simulink model "gm_inc_enc_v26"  (R2023a)
settings: Solver=FixedStepDiscrete  StartTime=0.0  StopTime=SimulationsDauer  RelTol=1e-3
undefined symbols (not defined in the file or in its folder): CW_CCW_Switch, d_axis_hit_CompareValue, DiscIntNeverNeededParam, f_ISR, IncPerTurn, inital_zero_speed_timeout, n_max, Offset_Position_elec, Offset_Position_mech, OmegaPerOverSampl, Periode, Phase_Delay_A, Phase_Delay_B, PolePair, QuadratureFactor, reciprocal_iterations, T_fpga, T_mech
libraries: hdlmdlgenlib x16, dspsrcs4 x3, dspswit3 x2, spsEdgeDetectorLib x2, simulink_extras x1
(part 1 of 3)
settings Model: Creator=Wendel_ELSYS  LastModifiedBy=ts
settings SolverCC: ConcurrentTasks=on  AlgebraicLoopSolver=TrustRegion  MinimalZcImpactIntegration=on
settings DataIOCC: LimitDataPoints=on  SaveFormat=Array
settings OptimizationCC: BlockReduction=off  ConditionallyExecuteInputs=off  DefaultParameterBehavior=Inlined  InheritOutputTypeSmallerThanSingle=on  ReuseModelBlockBuffer=off  LifeSpan=inf
settings DebuggingCC: ReadBeforeWriteMsg=DisableAll  WriteAfterWriteMsg=DisableAll  WriteAfterReadMsg=DisableAll  AlgebraicLoopMsg=error  InheritedTsInSrcMsg=none  SingleTaskRateTransMsg=error  ParameterOverflowMsg=none  UnconnectedInputMsg=warning  UnconnectedOutputMsg=warning  UnconnectedLineMsg=warning  SFUnexpectedBacktrackingDiag=warning  SFNoUnconditionalDefaultTransitionDiag=warning  SFExecutionAtInitializationDiag=none  ArithmeticOperatorsInVariantConditions=warning
settings HardwareCC: ProdBitPerPointer=32  ProdBitPerSizeT=32  ProdBitPerPtrDiffT=32  ProdLargestAtomicFloat=None  ProdIntDivRoundTo=Undefined  ProdEndianess=Unspecified  ProdWordSize=32  ProdHWDeviceType=ASIC/FPGA->ASIC/FPGA  ProdEqTarget=off
settings ModelReferenceCC: UpdateModelReferenceTargets=IfOutOfDate  EnableRefExpFcnMdlSchedulingChecks=on  PropagateSignalLabelsOutOfModel=off
settings SFSimCC: SFSimEcho=off  SimUseLocalCustomCode=off  CustomCodeUndefinedFunction=UseInterfaceOnly
settings RTWCC: RTWUseLocalCustomCode=off  DLArmComputeVersion=19.05
settings CodeAppCC: StateflowObjectComments=on
settings GRTTargetCC: TargetLangStandard=C89/C90 (ANSI)
settings ConfigComp: CovMetricSettings=dw  CovSaveCumulativeToWorkspaceVar=on  CovSaveSingleToWorkspaceVar=on  CovExternalEMLEnable=off
settings SimscapeCC: SimscapeNormalizeSystem=off

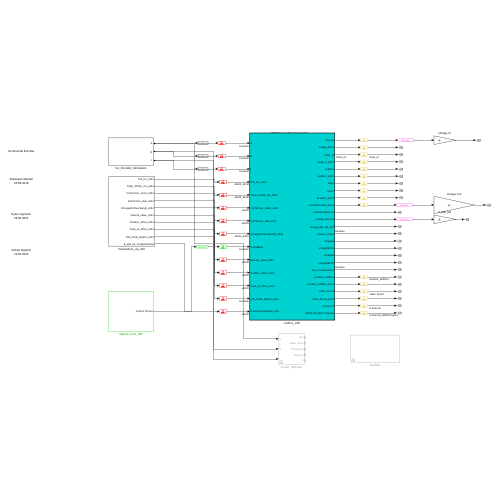
[thumbnail: Simulink's stored preview of the top-level diagram]
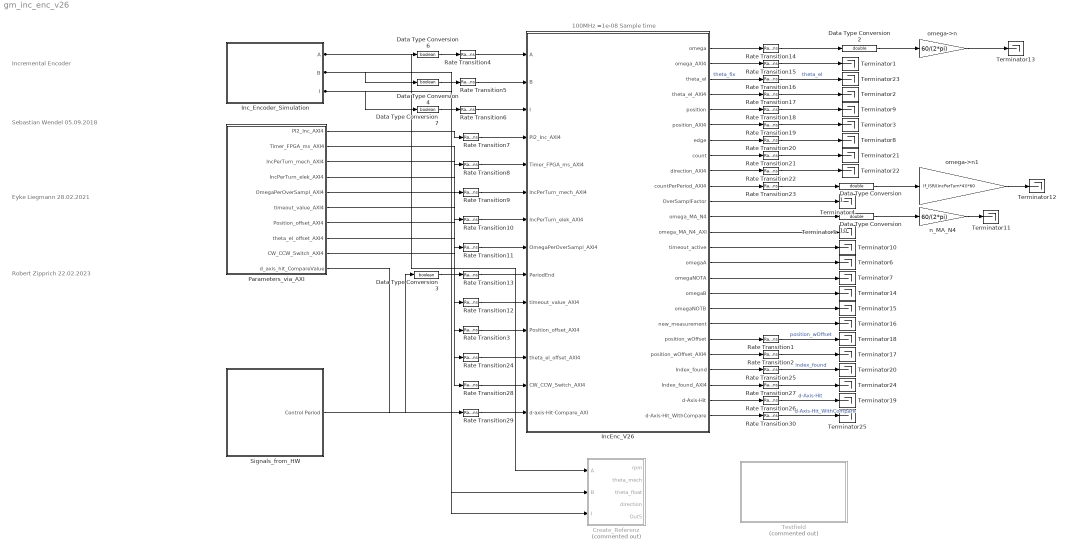
== system gm_inc_enc_v26 ==
  note: Robert Zipprich
      | 22.02.2023
  note: Eyke Liegmann
      | 28.02.2021
  note: Incremental Encoder
  note: Sebastian Wendel
      | 05.09.2018
  note: 100MHz =1e-08 Sample time
  Create_Referenz : Subsystem  Commented=on
  Data Type Conversion1 : DataTypeConversion  OutDataTypeStr=double  SaturateOnIntegerOverflow=off  RndMeth=Floor
  Data Type Conversion10 : DataTypeConversion  OutDataTypeStr=double  SaturateOnIntegerOverflow=off  RndMeth=Floor
  Data Type Conversion2 : DataTypeConversion  OutDataTypeStr=double  SaturateOnIntegerOverflow=off  RndMeth=Floor
  Data Type Conversion{3..4,6..7} (4 alike) : DataTypeConversion  OutDataTypeStr=boolean  SaturateOnIntegerOverflow=off  RndMeth=Floor
  IncEnc_V26 : Subsystem  TreatAsAtomicUnit=on
  Inc_Encoder_Simulation : Subsystem
  Parameters_via_AXI : Subsystem
  Rate Transition{1..2,14..23,25..27,30} (16 alike) : RateTransition  Deterministic=off  OutPortSampleTime=T_mech
  Rate Transition{3..13,24,28..29} (14 alike) : RateTransition  Deterministic=off  OutPortSampleTime=T_fpga
  Signals_from_HW : Subsystem
  Terminator{1..25} (25 alike) : Terminator
  Testfield : Subsystem  Commented=on
  n_MA_N4 : Gain  Gain=60/(2*pi)  OutDataTypeStr=double
  omega->n : Gain  Gain=60/(2*pi)  OutDataTypeStr=double
  omega->n1 : Gain  Gain=(f_ISR/(IncPerTurn*4))*60  OutDataTypeStr=double
  wires:
  Rate Transition30/1 -> Terminator25/1  "d-Axis-Hit_WithCompare"
  IncEnc_V26/25(d-Axis-Hit_WithCompare) -> Rate Transition30/1
  Parameters_via_AXI/10(d_axis_hit_CompareValue) -> Rate Transition29/1
  Rate Transition29/1 -> IncEnc_V26/14(d-axis-Hit-Compare_AXI)
  Parameters_via_AXI/9(CW_CCW_Switch_AXI4) -> Rate Transition28/1
  Rate Transition28/1 -> IncEnc_V26/13(CW_CCW_Switch_AXI4)
  IncEnc_V26/23(Index_found_AXI4) -> Rate Transition27/1
  Rate Transition27/1 -> Terminator24/1
  Rate Transition16/1 -> Terminator23/1  "theta_el"
  Rate Transition21/1 -> Terminator21/1
  Rate Transition22/1 -> Terminator22/1
  IncEnc_V26/24(d-Axis-Hit) -> Rate Transition26/1
  Rate Transition26/1 -> Terminator19/1  "d-Axis-Hit"
  Rate Transition25/1 -> Terminator20/1  "index_found"
  IncEnc_V26/22(Index_found) -> Rate Transition25/1
  Parameters_via_AXI/8(theta_el_offset_AXI4) -> Rate Transition24/1
  Rate Transition24/1 -> IncEnc_V26/12(theta_el_offset_AXI4)
  Parameters_via_AXI/7(Position_offset_AXI4) -> Rate Transition3/1
  Rate Transition3/1 -> IncEnc_V26/11(Position_offset_AXI4)
  IncEnc_V26/20(position_wOffset) -> Rate Transition1/1
  IncEnc_V26/21(position_wOffset_AXI4) -> Rate Transition2/1
  Rate Transition2/1 -> Terminator17/1
  Rate Transition1/1 -> Terminator18/1  "position_wOffset"
  Signals_from_HW/1(Control Period) -> Data Type Conversion3/1
  Inc_Encoder_Simulation/1(A) -> Create_Referenz/1(A), Data Type Conversion6/1
  Inc_Encoder_Simulation/3(I) -> Data Type Conversion7/1, Create_Referenz/3(I)
  Inc_Encoder_Simulation/2(B) -> Data Type Conversion4/1, Create_Referenz/2(B)
  Parameters_via_AXI/6(timeout_value_AXI4) -> Rate Transition12/1
  Parameters_via_AXI/5(OmegaPerOverSampl_AXI4) -> Rate Transition11/1
  Parameters_via_AXI/4(IncPerTurn_elek_AXI4) -> Rate Transition10/1
  Parameters_via_AXI/3(IncPerTurn_mech_AXI4) -> Rate Transition9/1
  Parameters_via_AXI/2(Timer_FPGA_ms_AXI4) -> Rate Transition8/1
  Parameters_via_AXI/1(PI2_Inc_AXI4) -> Rate Transition7/1
  IncEnc_V26/19(new_measurement) -> Terminator16/1
  IncEnc_V26/16(omegaNOTA) -> Terminator7/1
  IncEnc_V26/17(omegaB) -> Terminator14/1
  IncEnc_V26/18(omegaNOTB) -> Terminator15/1
  IncEnc_V26/15(omegaA) -> Terminator6/1
  omega->n1/1 -> Terminator12/1
  n_MA_N4/1 -> Terminator11/1
  Rate Transition18/1 -> Terminator9/1
  Rate Transition20/1 -> Terminator8/1
  IncEnc_V26/14(timeout_active) -> Terminator10/1
  Rate Transition12/1 -> IncEnc_V26/10(timeout_value_AXI4)
  Data Type Conversion10/1 -> n_MA_N4/1
  IncEnc_V26/13(omega_MA_N4_AXI) -> Terminator5/1
  IncEnc_V26/12(omega_MA_N4) -> Data Type Conversion10/1
  IncEnc_V26/11(OverSamplFactor) -> Terminator4/1
  Rate Transition23/1 -> Data Type Conversion1/1
  Rate Transition19/1 -> Terminator3/1
  Rate Transition17/1 -> Terminator2/1
  Rate Transition15/1 -> Terminator1/1
  Rate Transition14/1 -> Data Type Conversion2/1
  Rate Transition13/1 -> IncEnc_V26/9(PeriodEnd)
  Rate Transition11/1 -> IncEnc_V26/8(OmegaPerOverSampl_AXI4)
  Rate Transition10/1 -> IncEnc_V26/7(IncPerTurn_elek_AXI4)
  Rate Transition9/1 -> IncEnc_V26/6(IncPerTurn_mech_AXI4)
  Rate Transition8/1 -> IncEnc_V26/5(Timer_FPGA_ms_AXI4)
  Rate Transition7/1 -> IncEnc_V26/4(PI2_Inc_AXI4)
  Rate Transition6/1 -> IncEnc_V26/3(I)
  Rate Transition5/1 -> IncEnc_V26/2(B)
  Rate Transition4/1 -> IncEnc_V26/1(A)
  IncEnc_V26/6(position_AXI4) -> Rate Transition19/1
  Data Type Conversion3/1 -> Rate Transition13/1
  IncEnc_V26/10(countPerPeriod_AXI4) -> Rate Transition23/1
  Data Type Conversion1/1 -> omega->n1/1
  Data Type Conversion2/1 -> omega->n/1
  omega->n/1 -> Terminator13/1
  IncEnc_V26/2(omega_AXI4) -> Rate Transition15/1
  IncEnc_V26/4(theta_el_AXI4) -> Rate Transition17/1
  IncEnc_V26/5(position) -> Rate Transition18/1
  IncEnc_V26/3(theta_el) -> Rate Transition16/1  "theta_fix"
  IncEnc_V26/8(count) -> Rate Transition21/1
  IncEnc_V26/7(edge) -> Rate Transition20/1
  IncEnc_V26/9(direction_AXI4) -> Rate Transition22/1
  IncEnc_V26/1(omega) -> Rate Transition14/1
  Data Type Conversion7/1 -> Rate Transition6/1
  Data Type Conversion4/1 -> Rate Transition5/1
  Data Type Conversion6/1 -> Rate Transition4/1

== system gm_inc_enc_v26/Create_Referenz ==
  note: Überprüfen der Ausgabe:
      | (1/((Wert in Periodfelt von Counter)*Inkremente))*60
      | z.B. (1/((2.5*0.000001)*5000))*60
  A : Inport
  B : Inport  Port=2
  I : Inport  Port=3
  HardwareTimer_FPGA_in_ms*InCrements1 : Constant  Value=T_mech*IncPerTurn  OutDataTypeStr=double  SampleTime=T_mech
  IncrementalEncoder_Floating : Subsystem  Commented=on
  "daQuadraturEncoder " : Gain  Commented=on  Gain=4
  n_aus_theta : Subsystem  Commented=on  TreatAsAtomicUnit=on
  poles : Constant  Value=PolePair  OutDataTypeStr=uint8  SampleTime=T_mech
  rpm : Outport
  theta_mech : Outport  Port=2
  theta_float : Outport  Port=3
  direction : Outport  Port=4
  Out5 : Outport  Port=5
  wires:
  IncrementalEncoder_Floating/2(theta_mech) -> theta_mech/1
  "daQuadraturEncoder "/1 -> Out5/1
  IncrementalEncoder_Floating/1(rpm) -> rpm/1
  IncrementalEncoder_Floating/4(direction) -> direction/1
  HardwareTimer_FPGA_in_ms*InCrements1/1 -> n_aus_theta/2(T)
  I/1 -> IncrementalEncoder_Floating/3(I)
  poles/1 -> IncrementalEncoder_Floating/4(poles)
  IncrementalEncoder_Floating/3(theta_elec) -> theta_float/1  "theta_float"
  B/1 -> IncrementalEncoder_Floating/2(B)
  A/1 -> n_aus_theta/1(count), IncrementalEncoder_Floating/1(A)
  n_aus_theta/1(rpm) -> "daQuadraturEncoder "/1

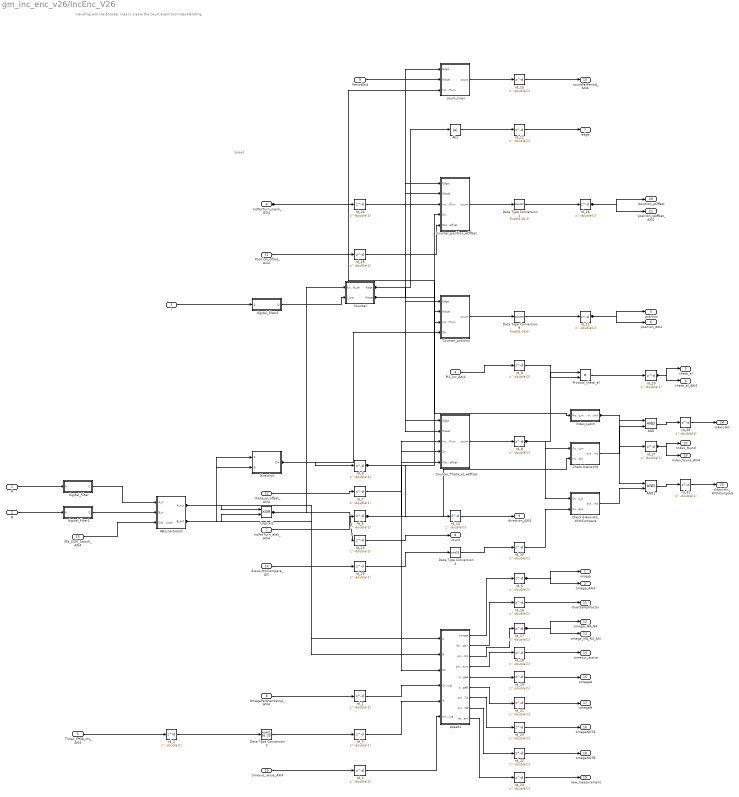
== system gm_inc_enc_v26/IncEnc_V26 ==
  note: Speed
  note: Handling with the Encoder lines to create the Count-Event and Index-Handling
  A : Inport  OutDataTypeStr=boolean  PortDimensions=1  SampleTime=1e-08
  B : Inport  Port=2  OutDataTypeStr=boolean  PortDimensions=1  SampleTime=1e-08
  I : Inport  Port=3  OutDataTypeStr=boolean  PortDimensions=1  SampleTime=1e-08
  PI2_Inc_AXI4 : Inport  Port=4  OutDataTypeStr=fixdt(0, 24, 24)  PortDimensions=1  SampleTime=1e-08
  Timer_FPGA_ms_AXI4 : Inport  Port=5  OutDataTypeStr=fixdt(0, 32, 32)  PortDimensions=1  SampleTime=1e-08
  IncPerTurn_mech_AXI4 : Inport  Port=6  OutDataTypeStr=uint16  PortDimensions=1  SampleTime=1e-08
  IncPerTurn_elek_AXI4 : Inport  Port=7  OutDataTypeStr=uint16  PortDimensions=1  SampleTime=1e-08
  OmegaPerOverSampl_AXI4 : Inport  Port=8  OutDataTypeStr=fixdt(1, 24, 11)  PortDimensions=1  SampleTime=1e-08
  PeriodEnd : Inport  Port=9  OutDataTypeStr=boolean  PortDimensions=1  SampleTime=1e-08
  timeout_value_AXI4 : Inport  Port=10  OutDataTypeStr=uint32  PortDimensions=1  SampleTime=1e-08
  Position_offset_AXI4 : Inport  Port=11  OutDataTypeStr=uint16  PortDimensions=1  SampleTime=1e-08
  theta_el_offset_AXI4 : Inport  Port=12  OutDataTypeStr=uint16  PortDimensions=1  SampleTime=1e-08
  CW_CCW_Switch_AXI4 : Inport  Port=13  OutDataTypeStr=boolean  PortDimensions=1  SampleTime=1e-08
  d-axis-Hit-Compare_AXI : Inport  Port=14  OutDataTypeStr=uint32  PortDimensions=1  SampleTime=1e-08
  AB-Line-Switch : Subsystem
  AND : Logic  AllPortsSameDT=off  OutDataTypeStr=boolean  SampleTime=1e-08
  AND1 : Logic  AllPortsSameDT=off  OutDataTypeStr=boolean  SampleTime=1e-08
  Abs : Abs  SampleTime=1e-08  OutDataTypeStr=fixdt(0, 1, 0)  RndMeth=Simplest  SaturateOnIntegerOverflow=off
  Check d-Axis-Hit : Subsystem
  Check d-Axis-Hit_WithCompare : Subsystem
  Counter : Subsystem
  Counter_Theta_el_wOffset : Subsystem
  Counter_position : Subsystem
  Counter_position_wOffset : Subsystem
  Data Type Conversion1 : DataTypeConversion  OutDataTypeStr=fixdt(0,16,0)
  Data Type Conversion3 : DataTypeConversion  OutDataTypeStr=fixdt(1, 38, 32)  SampleTime=1e-08  SaturateOnIntegerOverflow=off  RndMeth=Floor
  Data Type Conversion4 : DataTypeConversion  OutDataTypeStr=uint16  SampleTime=1e-08  SaturateOnIntegerOverflow=off  RndMeth=Floor
  Data Type Conversion9 : DataTypeConversion  OutDataTypeStr=fixdt(0,16,0)
  Direction : Subsystem
  Index_Latch : Subsystem
  Logical1 : Logic  Operator=XOR  AllPortsSameDT=off  OutDataTypeStr=boolean  SampleTime=1e-08
  Product_theta_el : Product  Inputs=**  OutDataTypeStr=fixdt(1, 24, 20)  SampleTime=1e-08
  count_lines : Subsystem
  digital_filter : Subsystem
  digital_filter1 : Subsystem
  digital_filter2 : Subsystem
  rd_0 : Delay  DelayLength=double(2)  InitialCondition=0  SampleTime=1e-08
  rd_{1..8,10..12,14..31} (29 alike) : Delay  DelayLength=double(1)  InitialCondition=0  SampleTime=1e-08
  rd_13 : Delay  DelayLength=double(2)  InitialCondition=0  SampleTime=1e-08
  rd_9 : Delay  DelayLength=double(2)  InitialCondition=0  SampleTime=1e-08
  speed1 : Subsystem
  omega : Outport  SampleTime=1e-08  VectorParamsAs1DForOutWhenUnconnected=off
  omega_AXI4 : Outport  Port=2  SampleTime=1e-08  VectorParamsAs1DForOutWhenUnconnected=off
  theta_el : Outport  Port=3  SampleTime=1e-08  VectorParamsAs1DForOutWhenUnconnected=off
  theta_el_AXI4 : Outport  Port=4  SampleTime=1e-08  VectorParamsAs1DForOutWhenUnconnected=off
  position : Outport  Port=5  SampleTime=1e-08  VectorParamsAs1DForOutWhenUnconnected=off
  position_AXI4 : Outport  Port=6  SampleTime=1e-08  VectorParamsAs1DForOutWhenUnconnected=off
  edge : Outport  Port=7  SampleTime=1e-08  VectorParamsAs1DForOutWhenUnconnected=off
  count : Outport  Port=8  SampleTime=1e-08  VectorParamsAs1DForOutWhenUnconnected=off
  direction_AXI4 : Outport  Port=9  SampleTime=1e-08  VectorParamsAs1DForOutWhenUnconnected=off
  countPerPeriod_AXI4 : Outport  Port=10  SampleTime=1e-08  VectorParamsAs1DForOutWhenUnconnected=off
  OverSamplFactor : Outport  Port=11  SampleTime=1e-08  VectorParamsAs1DForOutWhenUnconnected=off
  omega_MA_N4 : Outport  Port=12  SampleTime=1e-08  VectorParamsAs1DForOutWhenUnconnected=off
  omega_MA_N4_AXI : Outport  Port=13  SampleTime=1e-08  VectorParamsAs1DForOutWhenUnconnected=off
  timeout_active : Outport  Port=14  OutDataTypeStr=boolean  SampleTime=1e-08  VectorParamsAs1DForOutWhenUnconnected=off
  omegaA : Outport  Port=15  SampleTime=1e-08  VectorParamsAs1DForOutWhenUnconnected=off
  omegaNOTA : Outport  Port=16  SampleTime=1e-08  VectorParamsAs1DForOutWhenUnconnected=off
  omegaB : Outport  Port=17  SampleTime=1e-08  VectorParamsAs1DForOutWhenUnconnected=off
  omegaNOTB : Outport  Port=18  SampleTime=1e-08  VectorParamsAs1DForOutWhenUnconnected=off
  new_measurement : Outport  Port=19  OutDataTypeStr=boolean  SampleTime=1e-08  VectorParamsAs1DForOutWhenUnconnected=off
  position_wOffset : Outport  Port=20  SampleTime=1e-08  VectorParamsAs1DForOutWhenUnconnected=off
  position_wOffset_AXI4 : Outport  Port=21  SampleTime=1e-08  VectorParamsAs1DForOutWhenUnconnected=off
  Index_found : Outport  Port=22  SampleTime=1e-08  VectorParamsAs1DForOutWhenUnconnected=off
  Index_found_AXI4 : Outport  Port=23  SampleTime=1e-08  VectorParamsAs1DForOutWhenUnconnected=off
  d-Axis-Hit : Outport  Port=24  SampleTime=1e-08  VectorParamsAs1DForOutWhenUnconnected=off
  d-Axis-Hit_WithCompare : Outport  Port=25  SampleTime=1e-08  VectorParamsAs1DForOutWhenUnconnected=off
  wires:
  AB-Line-Switch/1(A_out) -> Logical1/1, speed1/1(A), Direction/1(A)
  AB-Line-Switch/2(B_out) -> Logical1/2, speed1/2(B), Direction/2(B)
  AND/1 -> rd_28/1
  AND1/1 -> rd_31/1
  Abs/1 -> rd_12/1
  Check d-Axis-Hit/1(d-axis-hit) -> AND/2
  Check d-Axis-Hit_WithCompare/1(d-axis-hit) -> AND1/2
  Counter/1(Edge) -> Abs/1, Counter_position/1(Edge), Counter_Theta_el_wOffset/1(Edge), Counter_position_wOffset/1(Edge), count_lines/1(Edge)
  Counter/2(Reset) -> Counter_position/2(Reset), Counter_Theta_el_wOffset/2(Reset), Counter_position_wOffset/2(Reset), Index_Latch/1(Reset_in)
  Counter_position/1(count) -> Data Type Conversion9/1
  Counter_position_wOffset/1(count) -> Data Type Conversion1/1
  Data Type Conversion3/1 -> rd_3/1
  Data Type Conversion4/1 -> rd_30/1
  Logical1/1 -> rd_13/1, Counter/1(Enable_ctr)
  count_lines/1(count) -> rd_15/1
  digital_filter/1(Q) -> AB-Line-Switch/1(A_in)
  digital_filter1/1(Q) -> AB-Line-Switch/2(B_in)
  digital_filter2/1(Q) -> Counter/2(I_line)
  speed1/2(OverSamplFactor) -> rd_16/1
  speed1/4(timeout_active) -> rd_18/1
  speed1/5(omegaA) -> rd_19/1
  speed1/6(omegaB) -> rd_21/1
  speed1/7(omegaNOTA) -> rd_20/1
  speed1/8(omegaNOTB) -> rd_22/1
  speed1/9(new_measurement) -> rd_23/1
  A/1 -> digital_filter/1(A)
  B/1 -> digital_filter1/1(A)
  I/1 -> digital_filter2/1(A)
  PI2_Inc_AXI4/1 -> rd_9/1
  Timer_FPGA_ms_AXI4/1 -> rd_2/1
  IncPerTurn_mech_AXI4/1 -> rd_24/1, Counter_position/3(IncsPerTurn), count_lines/3(IncsPerTurn)
  OmegaPerOverSampl_AXI4/1 -> rd_1/1
  PeriodEnd/1 -> count_lines/2(Reset)
  timeout_value_AXI4/1 -> rd_4/1
  Position_offset_AXI4/1 -> rd_25/1
  theta_el_offset_AXI4/1 -> rd_7/1
  CW_CCW_Switch_AXI4/1 -> AB-Line-Switch/3(CW_CCW_Switch)
  d-axis-Hit-Compare_AXI/1 -> rd_29/1
  rd_13/1 -> count/1
  rd_24/1 -> Counter_position_wOffset/3(IncsPerTurn)
  rd_15/1 -> countPerPeriod_AXI4/1
  rd_16/1 -> OverSamplFactor/1
  rd_18/1 -> timeout_active/1
  rd_19/1 -> omegaA/1
  rd_21/1 -> omegaB/1
  rd_20/1 -> omegaNOTA/1
  rd_22/1 -> omegaNOTB/1
  rd_23/1 -> new_measurement/1
  rd_28/1 -> d-Axis-Hit/1
  rd_31/1 -> d-Axis-Hit_WithCompare/1
  rd_12/1 -> edge/1
  rd_3/1 -> speed1/5(T)
  rd_30/1 -> Check d-Axis-Hit_WithCompare/2(Counter_Compare)
  rd_9/1 -> Product_theta_el/2
  rd_2/1 -> Data Type Conversion3/1
  rd_1/1 -> speed1/4(OmegaPerOverSampl)
  rd_4/1 -> speed1/6(timeout_value)
  rd_25/1 -> Counter_position_wOffset/5(Position_offset)
  rd_7/1 -> Counter_Theta_el_wOffset/5(Position_offset)
  rd_29/1 -> Data Type Conversion4/1
  Counter_Theta_el_wOffset/1(count) -> rd_8/1
  rd_8/1 -> Check d-Axis-Hit/1(Count_in), Check d-Axis-Hit_WithCompare/1(Count_in), Product_theta_el/1
  Data Type Conversion1/1 -> rd_26/1
  rd_26/1 -> position_wOffset_AXI4/1, position_wOffset/1
  Data Type Conversion9/1 -> rd_11/1
  rd_11/1 -> position/1, position_AXI4/1
  Direction/1(Dir) -> Counter_position/4(Dir), rd_0/1
  rd_0/1 -> Counter_position_wOffset/4(Dir), Counter_Theta_el_wOffset/4(Dir), speed1/3(Dir), rd_14/1
  rd_14/1 -> direction_AXI4/1
  Index_Latch/1(Index_found) -> AND/1, AND1/1, rd_27/1
  rd_27/1 -> Index_found/1, Index_found_AXI4/1
  Product_theta_el/1 -> rd_10/1
  rd_10/1 -> theta_el/1, theta_el_AXI4/1
  speed1/1(omega) -> rd_5/1
  rd_5/1 -> omega_AXI4/1, omega/1
  speed1/3(omega_MA_N4) -> rd_17/1
  rd_17/1 -> omega_MA_N4_AXI/1, omega_MA_N4/1
  IncPerTurn_elek_AXI4/1 -> rd_6/1
  rd_6/1 -> Check d-Axis-Hit/2(IncPerTurn_elek_AXI4), Counter_Theta_el_wOffset/3(IncsPerTurn)

== system gm_inc_enc_v26/Inc_Encoder_Simulation ==
  Logical Operator1 : Logic  Operator=XOR  AllPortsSameDT=off  OutDataTypeStr=boolean
  Manual Switch : ManualSwitch
  Manual Switch1 : ManualSwitch
  Manual Switch2 : ManualSwitch
  Pulse Generator1 0.1 : DiscretePulseGenerator  Commented=on  PulseType=Time based  Period=Periode  PulseWidth=50  PhaseDelay=Phase_Delay_B  SampleTime=T_mech  VectorParams1D=off
  Pulse Generator2 : DiscretePulseGenerator  Commented=on  PulseType=Time based  Period=Periode  PulseWidth=50  PhaseDelay=Phase_Delay_A  SampleTime=T_mech  VectorParams1D=off
  Rate Transition : RateTransition  Deterministic=off  OutPortSampleTime=T_mech
  Rate Transition2 : RateTransition  Deterministic=off  OutPortSampleTime=T_mech
  Signal From Workspace : dspsrcs4/Signal From Workspace  Commented=on  X=A_ila  Ts=T_mech  nsamps=1  OutputAfterFinalValue=Setting to zero  ignoreOrWarnInputAndFrameLengths=off  OutputFrames=off
  Signal From Workspace1 : dspsrcs4/Signal From Workspace  Commented=on  X=B_ila  Ts=T_mech  nsamps=1  OutputAfterFinalValue=Setting to zero  ignoreOrWarnInputAndFrameLengths=off  OutputFrames=off
  Signal From Workspace2 : dspsrcs4/Signal From Workspace  Commented=on  X=I_ila  Ts=T_mech  nsamps=1  OutputAfterFinalValue=Setting to zero  ignoreOrWarnInputAndFrameLengths=off  OutputFrames=off
  Simulate_I_Line : dspswit3/Counter  Direction=Up  CountEvent=Either edge  CounterSize=User defined  MaxCount=IncPerTurn*4  InitialCount=123  Output=Hit  HitValue=IncPerTurn*4  ResetInput=off  SamplesPerFrame=1  Ts=1  CntDtype=double  HitDtype=Boolean
  A : Outport
  B : Outport  Port=2
  I : Outport  Port=3
  wires:
  Manual Switch2/1 -> I/1  "I"
  Simulate_I_Line/1 -> Manual Switch2/1
  Signal From Workspace2/1 -> Manual Switch2/2
  Rate Transition2/1 -> Manual Switch1/1
  Rate Transition/1 -> Manual Switch/1
  Pulse Generator1 0.1/1 -> Rate Transition2/1  "B"
  Manual Switch/1 -> Logical Operator1/1, A/1
  Signal From Workspace/1 -> Manual Switch/2
  Manual Switch1/1 -> Logical Operator1/2, B/1
  Logical Operator1/1 -> Simulate_I_Line/1
  Signal From Workspace1/1 -> Manual Switch1/2
  Pulse Generator2/1 -> Rate Transition/1  "A"

== system gm_inc_enc_v26/Parameters_via_AXI ==
  CW_CCW_Switch_REG : Constant  Value=CW_CCW_Switch  OutDataTypeStr=boolean  SampleTime=T_mech
  CW_CCW_Switch_REG1 : Constant  Value=d_axis_hit_CompareValue  OutDataTypeStr=uint32  SampleTime=T_mech
  Constant : Constant  OutDataTypeStr=boolean
  Constant1 : Constant  Value=0  OutDataTypeStr=boolean
  "EncoderIncsPerTurn_elek_REG " : Constant  Value=(IncPerTurn*QuadratureFactor)/PolePair  OutDataTypeStr=fixdt(0,16,0)  SampleTime=T_mech
  EncoderIncsPerTurn_mech_REG : Constant  Value=IncPerTurn*QuadratureFactor  OutDataTypeStr=fixdt(0,16,0)  SampleTime=T_mech
  EncoderPI2_Inc_elek_REG : Constant  Value=(2*pi/(IncPerTurn*QuadratureFactor))*PolePair  OutDataTypeStr=fixdt(0,24,24)  SampleTime=T_mech
  Encoder_Time_REG HardwareTimer_FPGA_in_s*Increments and divide by 2PI for scaling to rad : Constant  Value=(T_fpga*IncPerTurn)/(2*pi)  OutDataTypeStr=fixdt(0,32,32)  SampleTime=T_mech
  Manual Switch : ManualSwitch  CurrentSetting=0
  Manual Switch1 : ManualSwitch  CurrentSetting=0
  OverSamplingFactorInverseREG : Constant  Value=OmegaPerOverSampl  OutDataTypeStr=fixdt(1,24,11)  SampleTime=T_mech
  Position_Offset_REG : Constant  Value=Offset_Position_mech  OutDataTypeStr=fixdt(0,16,0)  SampleTime=T_mech
  theta_el_Offset_REG : Constant  Value=Offset_Position_elec  OutDataTypeStr=fixdt(0,16,0)  SampleTime=T_mech
  zero_speed_timeout_REG : Constant  Value=inital_zero_speed_timeout  OutDataTypeStr=uint32  SampleTime=T_mech
  PI2_Inc_AXI4 : Outport
  Timer_FPGA_ms_AXI4 : Outport  Port=2
  IncPerTurn_mech_AXI4 : Outport  Port=3
  IncPerTurn_elek_AXI4 : Outport  Port=4
  OmegaPerOverSampl_AXI4 : Outport  Port=5
  timeout_value_AXI4 : Outport  Port=6
  Position_offset_AXI4 : Outport  Port=7
  theta_el_offset_AXI4 : Outport  Port=8
  CW_CCW_Switch_AXI4 : Outport  Port=9
  d_axis_hit_CompareValue : Outport  Port=10
  wires:
  CW_CCW_Switch_REG1/1 -> d_axis_hit_CompareValue/1
  Manual Switch1/1 -> CW_CCW_Switch_AXI4/1
  Manual Switch/1 -> Manual Switch1/2
  CW_CCW_Switch_REG/1 -> Manual Switch1/1
  Constant1/1 -> Manual Switch/2
  Constant/1 -> Manual Switch/1
  theta_el_Offset_REG/1 -> theta_el_offset_AXI4/1
  Position_Offset_REG/1 -> Position_offset_AXI4/1
  EncoderIncsPerTurn_mech_REG/1 -> IncPerTurn_mech_AXI4/1
  EncoderPI2_Inc_elek_REG/1 -> PI2_Inc_AXI4/1
  OverSamplingFactorInverseREG/1 -> OmegaPerOverSampl_AXI4/1
  zero_speed_timeout_REG/1 -> timeout_value_AXI4/1
  Encoder_Time_REG HardwareTimer_FPGA_in_s*Increments and divide by 2PI for scaling to rad/1 -> Timer_FPGA_ms_AXI4/1
  "EncoderIncsPerTurn_elek_REG "/1 -> IncPerTurn_elek_AXI4/1

== system gm_inc_enc_v26/Signals_from_HW ==
  uCTakt : DiscretePulseGenerator  PulseType=Time based  Period=1/f_ISR  PulseWidth=f_ISR*T_fpga *100  SampleTime=T_mech  VectorParams1D=off
  Control Period : Outport
  wires:
  uCTakt/1 -> Control Period/1  "Control Period"

== system gm_inc_enc_v26/Testfield ==
  Cast To Boolean1 : DataTypeConversion  OutDataTypeStr=boolean  SaturateOnIntegerOverflow=off  RndMeth=Floor
  Constant1 : Constant  Value=256*4
  Constant2 : Constant
  Constant3 : Constant  Value=512
  Counter_position_wOffset : Subsystem  TreatAsAtomicUnit=on
  Index_Latch : Subsystem
  Pulse Generator : DiscretePulseGenerator  Period=10  SampleTime=1/10e3
  Pulse Generator1 : DiscretePulseGenerator  Period=100000  PhaseDelay=42505  SampleTime=1/10e3
  Scope : Scope  NumInputPorts=3
  Scope1 : Scope  NumInputPorts=2
  wires:
  Index_Latch/1(Index_found) -> Scope1/2
  Counter_position_wOffset/1(count) -> Scope/3  "count_mech"
  Pulse Generator1/1 -> Cast To Boolean1/1
  Cast To Boolean1/1 -> Counter_position_wOffset/2(Reset), Index_Latch/1(Reset_in), Scope1/1, Scope/2
  Constant2/1 -> Counter_position_wOffset/4(Dir)
  Constant3/1 -> Counter_position_wOffset/5(Position_offset)
  Pulse Generator/1 -> Scope/1, Counter_position_wOffset/1(Edge)
  Constant1/1 -> Counter_position_wOffset/3(IncsPerTurn)

== system gm_inc_enc_v26/Create_Referenz/IncrementalEncoder_Floating ==
  A : Inport
  B : Inport  Port=2
  I : Inport  Port=3
  poles : Inport  Port=4
  Add : Sum  Inputs=+-  OutDataTypeStr=fixdt(1,16,0)
  Counter3 : dspswit3/Counter  Direction=Up  CountEvent=Either edge  CounterSize=User defined  MaxCount=IncPerTurn*4  InitialCount=0  Output=Count  HitValue=32  ResetInput=on  SamplesPerFrame=1  Ts=1  CntDtype=double  HitDtype=Logical
  CutTheta_0_2PI : Subsystem
  Edge Detector2 : spsEdgeDetectorLib/Edge Detector  model=Rising  ic=0  Ts=-1
  Edge Detector3 : spsEdgeDetectorLib/Edge Detector  model=Rising  ic=0  Ts=-1
  Logical Operator1 : Logic  Operator=XOR  AllPortsSameDT=off  OutDataTypeStr=boolean
  Logical Operator3 : Logic  AllPortsSameDT=off  OutDataTypeStr=boolean
  Logical Operator4 : Logic  Operator=NOT  AllPortsSameDT=off  OutDataTypeStr=boolean
  Logical Operator5 : Logic  AllPortsSameDT=off  OutDataTypeStr=boolean
  Logical Operator6 : Logic  Operator=NOT  AllPortsSameDT=off  OutDataTypeStr=boolean
  Product : Product
  S-R Flip-Flop1 : simulink_extras/Flip Flops/S-R Flip-Flop  initial_condition=0
  Scope1 : Scope  NumInputPorts=4
  cut_theta_2pi : Gain  Gain=(2*pi)/(IncPerTurn*QuadratureFactor)
  cut_theta_2pi1 : Gain  Gain=(2*pi)/(IncPerTurn*QuadratureFactor)
  n_aus_theta_v4 : Subsystem
  rpm : Outport  VectorParamsAs1DForOutWhenUnconnected=off
  theta_mech : Outport  Port=2  VectorParamsAs1DForOutWhenUnconnected=off
  theta_elec : Outport  Port=3  VectorParamsAs1DForOutWhenUnconnected=off
  direction : Outport  Port=4  VectorParamsAs1DForOutWhenUnconnected=off
  wires:
  Add/1 -> direction/1
  B/1 -> Logical Operator1/2, Logical Operator4/1, Edge Detector3/1
  A/1 -> Logical Operator1/1, Edge Detector2/1, Logical Operator6/1
  S-R Flip-Flop1/2 -> Add/2
  S-R Flip-Flop1/1 -> Add/1
  Logical Operator5/1 -> S-R Flip-Flop1/2
  Logical Operator6/1 -> Logical Operator5/2
  Edge Detector3/1 -> Logical Operator5/1
  Logical Operator3/1 -> S-R Flip-Flop1/1
  Logical Operator4/1 -> Logical Operator3/2
  Edge Detector2/1 -> Logical Operator3/1
  CutTheta_0_2PI/1(Out1) -> theta_elec/1
  cut_theta_2pi1/1 -> CutTheta_0_2PI/1(In1)
  poles/1 -> Product/2
  Product/1 -> cut_theta_2pi1/1
  cut_theta_2pi/1 -> theta_mech/1, n_aus_theta_v4/1(theta), Scope1/2
  Logical Operator1/1 -> Counter3/1, Scope1/4
  n_aus_theta_v4/1(n) -> rpm/1
  Counter3/1 -> Scope1/1, cut_theta_2pi/1, Product/1
  I/1 -> Counter3/2

== system gm_inc_enc_v26/Create_Referenz/n_aus_theta ==
  count : Inport
  T : Inport  Port=2
  1/rps->1/omega : Gain  Gain=1/(2*pi)  OutDataTypeStr=double
  Add : Sum  Inputs=+-
  Add1 : Sum
  Constant : Constant  Value=0  OutDataTypeStr=double  SampleTime=-1
  Constant1 : Constant  Value=0  OutDataTypeStr=double  SampleTime=-1
  Constant2 : Constant  Value=0  OutDataTypeStr=double  SampleTime=-1
  Divide1 : Product  Inputs=/
  ProtectOverflow_T_count : Switch  Threshold=50  SaturateOnIntegerOverflow=off  InputSameDT=off
  ProtectOverflow_rps : Switch  Threshold=50  OutDataTypeStr=double  SaturateOnIntegerOverflow=off  InputSameDT=off
  Scope1 : Scope  NumInputPorts=4
  Scope2 : Scope  NumInputPorts=4
  T_count : Delay  DelayLength=1
  T_count_switch : Switch  Criteria=u2 ~= 0  SaturateOnIntegerOverflow=off  InputSameDT=off
  count_old : Delay  DelayLength=1
  count_old_switch : Switch  Criteria=u2 ~= 0  SaturateOnIntegerOverflow=off  InputSameDT=off
  speed_old : Delay  DelayLength=1
  speed_old_switch : Switch  Criteria=u2 ~= 0  SaturateOnIntegerOverflow=off  InputSameDT=off
  rpm : Outport  VectorParamsAs1DForOutWhenUnconnected=off
  wires:
  Divide1/1 -> rpm/1
  1/rps->1/omega/1 -> Divide1/1
  T_count_switch/1 -> ProtectOverflow_T_count/3, ProtectOverflow_T_count/2, Scope1/2, ProtectOverflow_rps/2
  count/1 -> count_old_switch/1, Add/1
  Add1/1 -> T_count_switch/3, speed_old_switch/1, Scope2/2
  T_count/1 -> Add1/2, Scope1/4
  ProtectOverflow_T_count/1 -> T_count/1
  T/1 -> Add1/1, Scope2/4
  speed_old/1 -> speed_old_switch/3
  speed_old_switch/1 -> speed_old/1, Scope2/3, ProtectOverflow_rps/3
  Constant2/1 -> ProtectOverflow_rps/1
  ProtectOverflow_rps/1 -> Scope2/1, 1/rps->1/omega/1
  Constant1/1 -> ProtectOverflow_T_count/1
  Add/1 -> T_count_switch/2, Scope1/1, count_old_switch/2, speed_old_switch/2
  Constant/1 -> T_count_switch/1
  count_old/1 -> Add/2, count_old_switch/3
  count_old_switch/1 -> count_old/1

== system gm_inc_enc_v26/IncEnc_V26/AB-Line-Switch ==
  A_in : Inport  OutDataTypeStr=boolean  PortDimensions=1  SampleTime=1e-08
  B_in : Inport  Port=2  OutDataTypeStr=boolean  PortDimensions=1  SampleTime=1e-08
  CW_CCW_Switch : Inport  Port=3  OutDataTypeStr=boolean  PortDimensions=1  SampleTime=1e-08
  Switch : Switch  Criteria=u2 > Threshold  Threshold=double(0)  OutDataTypeStr=boolean  SampleTime=1e-08  SaturateOnIntegerOverflow=off  InputSameDT=off
  Switch1 : Switch  Criteria=u2 > Threshold  Threshold=double(0)  OutDataTypeStr=boolean  SampleTime=1e-08  SaturateOnIntegerOverflow=off  InputSameDT=off
  rd_0 : Delay  DelayLength=double(1)  InitialCondition=0  SampleTime=1e-08
  A_out : Outport  SampleTime=1e-08
  B_out : Outport  Port=2  SampleTime=1e-08
  wires:
  A_in/1 -> Switch1/1, Switch/3
  B_in/1 -> Switch1/3, Switch/1
  Switch/1 -> A_out/1
  Switch1/1 -> B_out/1
  CW_CCW_Switch/1 -> rd_0/1
  rd_0/1 -> Switch/2, Switch1/2

== system gm_inc_enc_v26/IncEnc_V26/Check d-Axis-Hit ==
  Count_in : Inport  OutDataTypeStr=uint16  PortDimensions=1  SampleTime=1e-08
  IncPerTurn_elek_AXI4 : Inport  Port=2  OutDataTypeStr=uint16  PortDimensions=1  SampleTime=1e-08
  Constant : Constant  Value=0  OutDataTypeStr=uint16  SampleTime=1e-08
  Equal : RelationalOperator  Operator===  OutDataTypeStr=boolean  SampleTime=1e-08  InputSameDT=off
  Equal1 : RelationalOperator  Operator===  OutDataTypeStr=boolean  SampleTime=1e-08  InputSameDT=off
  OR : Logic  Operator=OR  AllPortsSameDT=off  OutDataTypeStr=boolean  SampleTime=1e-08
  d-axis-hit : Outport  SampleTime=1e-08  VectorParamsAs1DForOutWhenUnconnected=off
  wires:
  Count_in/1 -> Equal1/1, Equal/1
  IncPerTurn_elek_AXI4/1 -> Equal1/2
  Constant/1 -> Equal/2
  Equal/1 -> OR/1
  Equal1/1 -> OR/2
  OR/1 -> d-axis-hit/1

== system gm_inc_enc_v26/IncEnc_V26/Check d-Axis-Hit_WithCompare ==
  Count_in : Inport  OutDataTypeStr=uint16  PortDimensions=1  SampleTime=1e-08
  Counter_Compare : Inport  Port=2  OutDataTypeStr=uint16  PortDimensions=1  SampleTime=1e-08
  Equal : RelationalOperator  Operator===  OutDataTypeStr=boolean  SampleTime=1e-08  InputSameDT=off
  d-axis-hit : Outport  SampleTime=1e-08  VectorParamsAs1DForOutWhenUnconnected=off
  wires:
  Count_in/1 -> Equal/1
  Counter_Compare/1 -> Equal/2
  Equal/1 -> d-axis-hit/1

== system gm_inc_enc_v26/IncEnc_V26/Counter ==
  note: Reset
  note: 1 for one cycle if edge recognized
  Enable_ctr : Inport  OutDataTypeStr=boolean  PortDimensions=1  SampleTime=1e-08
  I_line : Inport  Port=2  OutDataTypeStr=boolean  PortDimensions=1  SampleTime=1e-08
  Detec_edge : Sum  Inputs=+-  AccumDataTypeStr=int8  OutDataTypeStr=int8  SampleTime=1e-08
  Reset_flag : Sum  Inputs=+-  AccumDataTypeStr=uint8  OutDataTypeStr=uint8  SampleTime=1e-08
  rd_0 : Delay  DelayLength=double(1)  InitialCondition=0  SampleTime=1e-08
  rd_1 : Delay  DelayLength=double(1)  InitialCondition=0  SampleTime=1e-08
  rd_2 : Delay  DelayLength=double(1)  InitialCondition=0  SampleTime=1e-08
  reset_old_switch : Switch  Criteria=u2 ~= 0  Threshold=double(0)  OutDataTypeStr=boolean  SampleTime=1e-08  SaturateOnIntegerOverflow=off  InputSameDT=off
  reset_old_switch1 : Switch  Criteria=u2 ~= 0  Threshold=double(0)  OutDataTypeStr=boolean  SampleTime=1e-08  SaturateOnIntegerOverflow=off  InputSameDT=off
  Edge : Outport  SampleTime=1e-08  VectorParamsAs1DForOutWhenUnconnected=off
  Reset : Outport  Port=2  SampleTime=1e-08  VectorParamsAs1DForOutWhenUnconnected=off
  wires:
  I_line/1 -> Reset_flag/1, reset_old_switch/1
  Detec_edge/1 -> Edge/1, reset_old_switch1/2
  Reset_flag/1 -> Reset/1, reset_old_switch/2
  Enable_ctr/1 -> rd_0/1
  rd_0/1 -> reset_old_switch1/1, Detec_edge/1
  reset_old_switch1/1 -> rd_1/1
  rd_1/1 -> Detec_edge/2, reset_old_switch1/3
  reset_old_switch/1 -> rd_2/1
  rd_2/1 -> Reset_flag/2, reset_old_switch/3

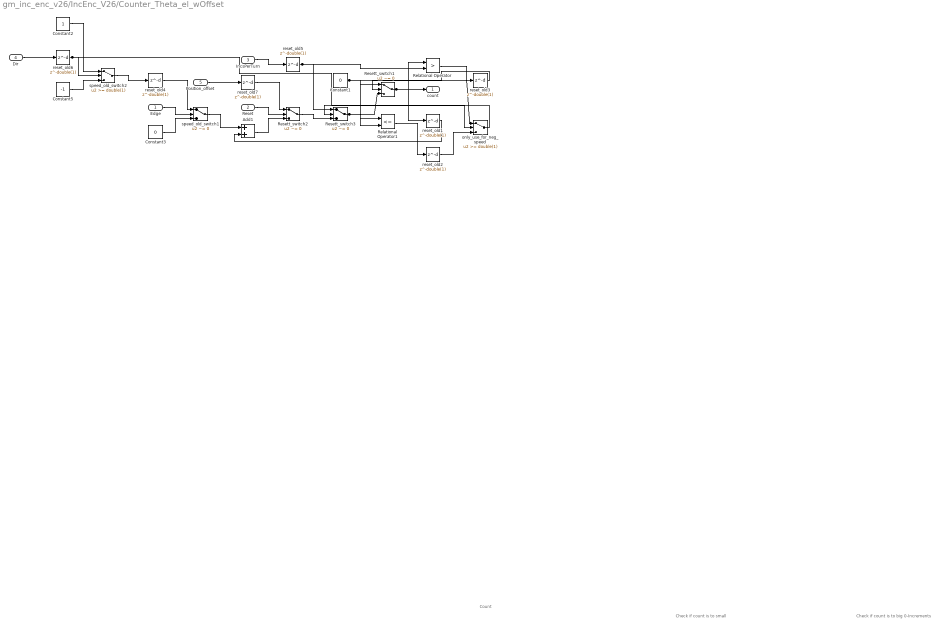
== system gm_inc_enc_v26/IncEnc_V26/Counter_Theta_el_wOffset ==
  note: Check if count is to small
  note: Count
  note: Check if count is to big 0-Increments
  Edge : Inport  OutDataTypeStr=int8  PortDimensions=1  SampleTime=1e-08
  Reset : Inport  Port=2  OutDataTypeStr=uint8  PortDimensions=1  SampleTime=1e-08
  IncsPerTurn : Inport  Port=3  OutDataTypeStr=uint16  PortDimensions=1  SampleTime=1e-08
  Dir : Inport  Port=4  OutDataTypeStr=fixdt(1, 4, 0)  PortDimensions=1  SampleTime=1e-08
  Position_offset : Inport  Port=5  OutDataTypeStr=uint16  PortDimensions=1  SampleTime=1e-08
  Add1 : Sum  AccumDataTypeStr=int16  OutDataTypeStr=int16  SampleTime=1e-08
  Constant1 : Constant  Value=0  OutDataTypeStr=int16  SampleTime=1e-08
  Constant2 : Constant  OutDataTypeStr=int16  SampleTime=1e-08
  Constant3 : Constant  Value=0  OutDataTypeStr=int16  SampleTime=1e-08
  Constant5 : Constant  Value=-1  OutDataTypeStr=int16  SampleTime=1e-08
  Relational Operator : RelationalOperator  Operator=>  OutDataTypeStr=boolean  SampleTime=1e-08  InputSameDT=off
  Relational Operator1 : RelationalOperator  Operator=<=  OutDataTypeStr=boolean  SampleTime=1e-08  InputSameDT=off
  Resett_switch1 : Switch  Criteria=u2 ~= 0  Threshold=double(0)  OutDataTypeStr=uint16  SampleTime=1e-08  SaturateOnIntegerOverflow=off  InputSameDT=off
  Resett_switch2 : Switch  Criteria=u2 ~= 0  Threshold=double(0)  OutDataTypeStr=int16  SampleTime=1e-08  SaturateOnIntegerOverflow=off  InputSameDT=off
  Resett_switch3 : Switch  Criteria=u2 ~= 0  Threshold=double(0)  OutDataTypeStr=int16  SampleTime=1e-08  SaturateOnIntegerOverflow=off  InputSameDT=off
  only_use_for_neg_speed : Switch  Threshold=double(1)  OutDataTypeStr=int16  SampleTime=1e-08  SaturateOnIntegerOverflow=off  InputSameDT=off
  reset_old{1..7} (7 alike) : Delay  DelayLength=double(1)  InitialCondition=0  SampleTime=1e-08
  speed_old_switch1 : Switch  Criteria=u2 ~= 0  Threshold=double(0)  OutDataTypeStr=int16  SampleTime=1e-08  SaturateOnIntegerOverflow=off  InputSameDT=off
  speed_old_switch2 : Switch  Threshold=double(1)  OutDataTypeStr=int16  SampleTime=1e-08  SaturateOnIntegerOverflow=off  InputSameDT=off
  count : Outport  SampleTime=1e-08  VectorParamsAs1DForOutWhenUnconnected=off
  wires:
  Edge/1 -> speed_old_switch1/2
  Reset/1 -> Resett_switch2/2
  IncsPerTurn/1 -> reset_old5/1
  Dir/1 -> reset_old6/1
  Position_offset/1 -> reset_old7/1
  Constant1/1 -> only_use_for_neg_speed/1, Resett_switch1/1, Relational Operator1/2
  Constant2/1 -> speed_old_switch2/1
  Constant3/1 -> speed_old_switch1/3
  Constant5/1 -> speed_old_switch2/3
  Resett_switch1/1 -> count/1, Relational Operator/1, reset_old1/1
  reset_old4/1 -> speed_old_switch1/1
  reset_old5/1 -> Resett_switch3/1, Relational Operator/2
  reset_old6/1 -> speed_old_switch2/2, only_use_for_neg_speed/2
  reset_old7/1 -> Resett_switch2/1
  speed_old_switch1/1 -> Add1/1
  speed_old_switch2/1 -> reset_old4/1
  Resett_switch2/1 -> Resett_switch3/3
  Add1/1 -> Resett_switch2/3
  reset_old1/1 -> Add1/2
  Relational Operator1/1 -> reset_old2/1
  reset_old2/1 -> only_use_for_neg_speed/3
  only_use_for_neg_speed/1 -> Resett_switch3/2
  Resett_switch3/1 -> Resett_switch1/3, Relational Operator1/1
  Relational Operator/1 -> reset_old3/1
  reset_old3/1 -> Resett_switch1/2

== system gm_inc_enc_v26/IncEnc_V26/Counter_position ==
  note: Check if count is to small
  note: Check if count is to big 0-Increments
  note: Count
  Edge : Inport  OutDataTypeStr=int8  PortDimensions=1  SampleTime=1e-08
  Reset : Inport  Port=2  OutDataTypeStr=uint8  PortDimensions=1  SampleTime=1e-08
  IncsPerTurn : Inport  Port=3  OutDataTypeStr=uint16  PortDimensions=1  SampleTime=1e-08
  Dir : Inport  Port=4  OutDataTypeStr=fixdt(1, 4, 0)  PortDimensions=1  SampleTime=1e-08
  Add1 : Sum  AccumDataTypeStr=int16  OutDataTypeStr=int16  SampleTime=1e-08
  Constant1 : Constant  Value=0  OutDataTypeStr=int16  SampleTime=1e-08
  Constant2 : Constant  OutDataTypeStr=int16  SampleTime=1e-08
  Constant3 : Constant  Value=0  OutDataTypeStr=int16  SampleTime=1e-08
  Constant4 : Constant  Value=0  OutDataTypeStr=int16  SampleTime=1e-08
  Constant5 : Constant  Value=-1  OutDataTypeStr=int16  SampleTime=1e-08
  Relational Operator : RelationalOperator  Operator=>  OutDataTypeStr=boolean  SampleTime=1e-08  InputSameDT=off
  Relational Operator1 : RelationalOperator  Operator=<=  OutDataTypeStr=boolean  SampleTime=1e-08  InputSameDT=off
  Resett_switch1 : Switch  Criteria=u2 ~= 0  Threshold=double(0)  OutDataTypeStr=uint16  SampleTime=1e-08  SaturateOnIntegerOverflow=off  InputSameDT=off
  Resett_switch2 : Switch  Criteria=u2 ~= 0  Threshold=double(0)  OutDataTypeStr=int16  SampleTime=1e-08  SaturateOnIntegerOverflow=off  InputSameDT=off
  Resett_switch3 : Switch  Criteria=u2 ~= 0  Threshold=double(0)  OutDataTypeStr=int16  SampleTime=1e-08  SaturateOnIntegerOverflow=off  InputSameDT=off
  only_use_for_neg_speed : Switch  Threshold=double(1)  OutDataTypeStr=int16  SampleTime=1e-08  SaturateOnIntegerOverflow=off  InputSameDT=off
  rd_0 : Delay  DelayLength=double(2)  InitialCondition=0  SampleTime=1e-08
  rd_{1,3..5} (4 alike) : Delay  DelayLength=double(1)  InitialCondition=0  SampleTime=1e-08
  rd_2 : Delay  DelayLength=double(3)  InitialCondition=0  SampleTime=1e-08
  speed_old_switch1 : Switch  Criteria=u2 ~= 0  Threshold=double(0)  OutDataTypeStr=int16  SampleTime=1e-08  SaturateOnIntegerOverflow=off  InputSameDT=off
  speed_old_switch2 : Switch  Threshold=double(1)  OutDataTypeStr=int16  SampleTime=1e-08  SaturateOnIntegerOverflow=off  InputSameDT=off
  count : Outport  SampleTime=1e-08  VectorParamsAs1DForOutWhenUnconnected=off
  wires:
  Edge/1 -> speed_old_switch1/2
  Reset/1 -> Resett_switch2/2
  Constant1/1 -> Resett_switch2/1
  Constant2/1 -> speed_old_switch2/1
  Constant3/1 -> speed_old_switch1/3
  Constant4/1 -> Relational Operator1/2, Resett_switch1/1, only_use_for_neg_speed/1
  Constant5/1 -> speed_old_switch2/3
  speed_old_switch1/1 -> Add1/1
  speed_old_switch2/1 -> rd_3/1
  Resett_switch2/1 -> Resett_switch3/3
  Add1/1 -> Resett_switch2/3
  Relational Operator1/1 -> rd_4/1
  only_use_for_neg_speed/1 -> Resett_switch3/2
  Resett_switch3/1 -> Resett_switch1/3, Relational Operator1/1
  Relational Operator/1 -> Resett_switch1/2
  rd_4/1 -> only_use_for_neg_speed/3
  rd_3/1 -> speed_old_switch1/1
  IncsPerTurn/1 -> rd_0/1
  rd_0/1 -> Resett_switch3/1, rd_1/1
  rd_1/1 -> Relational Operator/2
  Dir/1 -> rd_2/1
  rd_2/1 -> only_use_for_neg_speed/2, speed_old_switch2/2
  Resett_switch1/1 -> count/1, rd_5/1
  rd_5/1 -> Add1/2, Relational Operator/1

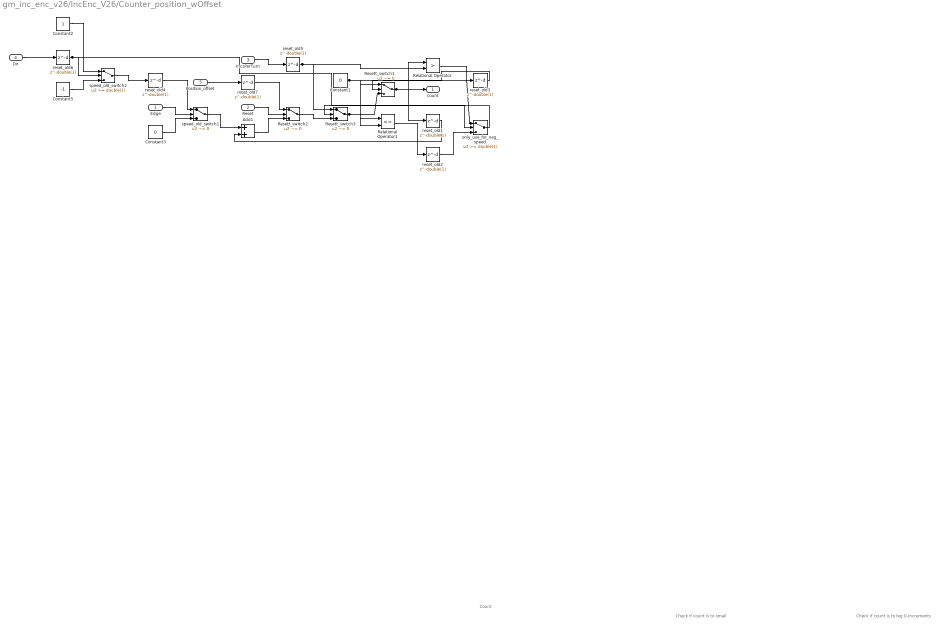
== system gm_inc_enc_v26/IncEnc_V26/Counter_position_wOffset ==
  note: Check if count is to big 0-Increments
  note: Count
  note: Check if count is to small
  Edge : Inport  OutDataTypeStr=int8  PortDimensions=1  SampleTime=1e-08
  Reset : Inport  Port=2  OutDataTypeStr=uint8  PortDimensions=1  SampleTime=1e-08
  IncsPerTurn : Inport  Port=3  OutDataTypeStr=uint16  PortDimensions=1  SampleTime=1e-08
  Dir : Inport  Port=4  OutDataTypeStr=fixdt(1, 4, 0)  PortDimensions=1  SampleTime=1e-08
  Position_offset : Inport  Port=5  OutDataTypeStr=uint16  PortDimensions=1  SampleTime=1e-08
  Add1 : Sum  AccumDataTypeStr=int16  OutDataTypeStr=int16  SampleTime=1e-08
  Constant1 : Constant  Value=0  OutDataTypeStr=int16  SampleTime=1e-08
  Constant2 : Constant  OutDataTypeStr=int16  SampleTime=1e-08
  Constant3 : Constant  Value=0  OutDataTypeStr=int16  SampleTime=1e-08
  Constant5 : Constant  Value=-1  OutDataTypeStr=int16  SampleTime=1e-08
  Relational Operator : RelationalOperator  Operator=>  OutDataTypeStr=boolean  SampleTime=1e-08  InputSameDT=off
  Relational Operator1 : RelationalOperator  Operator=<=  OutDataTypeStr=boolean  SampleTime=1e-08  InputSameDT=off
  Resett_switch1 : Switch  Criteria=u2 ~= 0  Threshold=double(0)  OutDataTypeStr=uint16  SampleTime=1e-08  SaturateOnIntegerOverflow=off  InputSameDT=off
  Resett_switch2 : Switch  Criteria=u2 ~= 0  Threshold=double(0)  OutDataTypeStr=int16  SampleTime=1e-08  SaturateOnIntegerOverflow=off  InputSameDT=off
  Resett_switch3 : Switch  Criteria=u2 ~= 0  Threshold=double(0)  OutDataTypeStr=int16  SampleTime=1e-08  SaturateOnIntegerOverflow=off  InputSameDT=off
  only_use_for_neg_speed : Switch  Threshold=double(1)  OutDataTypeStr=int16  SampleTime=1e-08  SaturateOnIntegerOverflow=off  InputSameDT=off
  reset_old{1..7} (7 alike) : Delay  DelayLength=double(1)  InitialCondition=0  SampleTime=1e-08
  speed_old_switch1 : Switch  Criteria=u2 ~= 0  Threshold=double(0)  OutDataTypeStr=int16  SampleTime=1e-08  SaturateOnIntegerOverflow=off  InputSameDT=off
  speed_old_switch2 : Switch  Threshold=double(1)  OutDataTypeStr=int16  SampleTime=1e-08  SaturateOnIntegerOverflow=off  InputSameDT=off
  count : Outport  SampleTime=1e-08  VectorParamsAs1DForOutWhenUnconnected=off
  wires:
  reset_old3/1 -> Resett_switch1/2
  Relational Operator/1 -> reset_old3/1
  Resett_switch3/1 -> Relational Operator1/1, Resett_switch1/3
  only_use_for_neg_speed/1 -> Resett_switch3/2
  reset_old2/1 -> only_use_for_neg_speed/3
  Relational Operator1/1 -> reset_old2/1
  reset_old1/1 -> Add1/2
  Add1/1 -> Resett_switch2/3
  Resett_switch2/1 -> Resett_switch3/3
  speed_old_switch2/1 -> reset_old4/1
  speed_old_switch1/1 -> Add1/1
  reset_old7/1 -> Resett_switch2/1
  reset_old6/1 -> only_use_for_neg_speed/2, speed_old_switch2/2
  reset_old5/1 -> Relational Operator/2, Resett_switch3/1
  reset_old4/1 -> speed_old_switch1/1
  Resett_switch1/1 -> reset_old1/1, Relational Operator/1, count/1
  Constant5/1 -> speed_old_switch2/3
  Constant3/1 -> speed_old_switch1/3
  Constant2/1 -> speed_old_switch2/1
  Constant1/1 -> Relational Operator1/2, Resett_switch1/1, only_use_for_neg_speed/1
  Position_offset/1 -> reset_old7/1
  Dir/1 -> reset_old6/1
  IncsPerTurn/1 -> reset_old5/1
  Reset/1 -> Resett_switch2/2
  Edge/1 -> speed_old_switch1/2

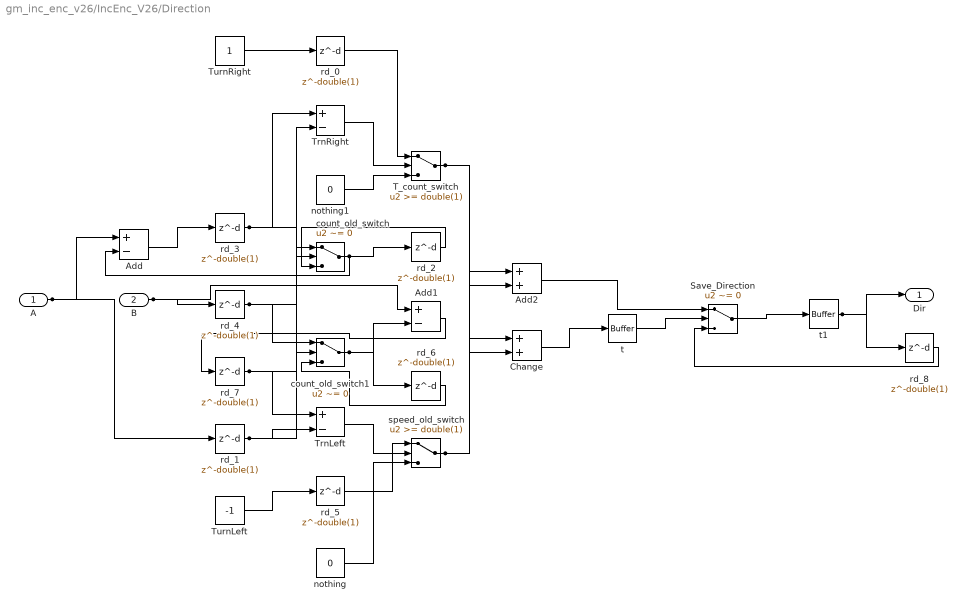
== system gm_inc_enc_v26/IncEnc_V26/Direction ==
  A : Inport  OutDataTypeStr=boolean  PortDimensions=1  SampleTime=1e-08
  B : Inport  Port=2  OutDataTypeStr=boolean  PortDimensions=1  SampleTime=1e-08
  Add : Sum  Inputs=+-  AccumDataTypeStr=fixdt(1, 4, 0)  OutDataTypeStr=fixdt(1, 4, 0)  SampleTime=1e-08
  Add1 : Sum  Inputs=+-  AccumDataTypeStr=fixdt(1, 4, 0)  OutDataTypeStr=fixdt(1, 4, 0)  SampleTime=1e-08
  Add2 : Sum  AccumDataTypeStr=fixdt(1, 4, 0)  OutDataTypeStr=fixdt(1, 4, 0)  SampleTime=1e-08
  Change : Sum  AccumDataTypeStr=fixdt(1, 4, 0)  OutDataTypeStr=fixdt(1, 4, 0)  SampleTime=1e-08
  Save_Direction : Switch  Criteria=u2 ~= 0  Threshold=double(0)  OutDataTypeStr=fixdt(1, 4, 0)  SampleTime=1e-08  SaturateOnIntegerOverflow=off  InputSameDT=off
  T_count_switch : Switch  Threshold=double(1)  OutDataTypeStr=fixdt(1, 4, 0)  SampleTime=1e-08  SaturateOnIntegerOverflow=off  InputSameDT=off
  TrnLeft : Sum  Inputs=+-  AccumDataTypeStr=fixdt(1, 4, 0)  OutDataTypeStr=fixdt(1, 4, 0)  SampleTime=1e-08
  TrnRight : Sum  Inputs=+-  AccumDataTypeStr=fixdt(1, 4, 0)  OutDataTypeStr=fixdt(1, 4, 0)  SampleTime=1e-08
  TurnLeft : Constant  Value=-1  OutDataTypeStr=fixdt(1, 4, 0)  SampleTime=1e-08
  TurnRight : Constant  OutDataTypeStr=fixdt(1, 4, 0)  SampleTime=1e-08
  count_old_switch : Switch  Criteria=u2 ~= 0  Threshold=double(0)  OutDataTypeStr=boolean  SampleTime=1e-08  SaturateOnIntegerOverflow=off  InputSameDT=off
  count_old_switch1 : Switch  Criteria=u2 ~= 0  Threshold=double(0)  OutDataTypeStr=boolean  SampleTime=1e-08  SaturateOnIntegerOverflow=off  InputSameDT=off
  nothing : Constant  Value=0  OutDataTypeStr=fixdt(1, 4, 0)  SampleTime=1e-08
  nothing1 : Constant  Value=0  OutDataTypeStr=fixdt(1, 4, 0)  SampleTime=1e-08
  rd_{0..8} (9 alike) : Delay  DelayLength=double(1)  InitialCondition=0  SampleTime=1e-08
  speed_old_switch : Switch  Threshold=double(1)  OutDataTypeStr=fixdt(1, 4, 0)  SampleTime=1e-08  SaturateOnIntegerOverflow=off  InputSameDT=off
  t : hdlmdlgenlib/Buffer
  t1 : hdlmdlgenlib/Buffer
  Dir : Outport  SampleTime=1e-08  VectorParamsAs1DForOutWhenUnconnected=off
  wires:
  Add2/1 -> Save_Direction/1
  Change/1 -> t/1
  t/1 -> Save_Direction/2
  T_count_switch/1 -> Change/1, Add2/1
  TrnLeft/1 -> speed_old_switch/2
  TrnRight/1 -> T_count_switch/2
  TurnLeft/1 -> rd_5/1
  TurnRight/1 -> rd_0/1
  t1/1 -> rd_8/1, Dir/1
  nothing/1 -> speed_old_switch/3
  nothing1/1 -> T_count_switch/3
  speed_old_switch/1 -> Change/2, Add2/2
  count_old_switch/1 -> rd_2/1, Add/2
  count_old_switch1/1 -> rd_6/1, Add1/2
  Save_Direction/1 -> t1/1
  rd_5/1 -> speed_old_switch/1
  rd_0/1 -> T_count_switch/1
  rd_2/1 -> count_old_switch/3
  rd_8/1 -> Save_Direction/3
  rd_6/1 -> count_old_switch1/3
  A/1 -> Add/1, rd_1/1
  rd_1/1 -> count_old_switch/1, TrnLeft/2
  B/1 -> Add1/1, rd_4/1
  rd_4/1 -> TrnRight/2, count_old_switch1/1
  Add/1 -> rd_3/1
  rd_3/1 -> count_old_switch/2, TrnRight/1
  Add1/1 -> rd_7/1
  rd_7/1 -> count_old_switch1/2, TrnLeft/1

== system gm_inc_enc_v26/IncEnc_V26/Index_Latch ==
  Reset_in : Inport  OutDataTypeStr=uint8  PortDimensions=1  SampleTime=1e-08
  Constant : Constant  OutDataTypeStr=boolean  SampleTime=1e-08
  Constant4 : Constant  Value=0  OutDataTypeStr=boolean  SampleTime=1e-08
  OR : Logic  Operator=OR  AllPortsSameDT=off  OutDataTypeStr=boolean  SampleTime=1e-08
  Switch : Switch  Criteria=u2 > Threshold  Threshold=double(0)  OutDataTypeStr=boolean  SampleTime=1e-08  SaturateOnIntegerOverflow=off  InputSameDT=off
  rd_0 : Delay  DelayLength=double(1)  InitialCondition=0  SampleTime=1e-08
  Index_found : Outport  SampleTime=1e-08
  wires:
  Reset_in/1 -> OR/1
  Constant/1 -> Switch/1
  Constant4/1 -> Switch/3
  Switch/1 -> rd_0/1, Index_found/1
  OR/1 -> Switch/2
  rd_0/1 -> OR/2

== system gm_inc_enc_v26/IncEnc_V26/count_lines ==
  note: Count
  note: Check if count is to big in order to safe for value overflow
  note: Set new counter value
  Edge : Inport  OutDataTypeStr=int8  PortDimensions=1  SampleTime=1e-08
  Reset : Inport  Port=2  OutDataTypeStr=boolean  PortDimensions=1  SampleTime=1e-08
  IncsPerTurn : Inport  Port=3  OutDataTypeStr=uint16  PortDimensions=1  SampleTime=1e-08
  Add1 : Sum  AccumDataTypeStr=int16  OutDataTypeStr=int16  SampleTime=1e-08
  Constant1 : Constant  Value=0  OutDataTypeStr=int16  SampleTime=1e-08
  Constant2 : Constant  OutDataTypeStr=int16  SampleTime=1e-08
  Constant3 : Constant  Value=0  OutDataTypeStr=int16  SampleTime=1e-08
  Constant4 : Constant  Value=10  OutDataTypeStr=int16  SampleTime=1e-08
  Relational Operator : RelationalOperator  Operator=>  OutDataTypeStr=boolean  SampleTime=1e-08  InputSameDT=off
  Reset_when_overflow : Sum  AccumDataTypeStr=fixdt(1, 18, 0)  OutDataTypeStr=int16  SampleTime=1e-08
  Resett_switch1 : Switch  Criteria=u2 ~= 0  Threshold=double(0)  OutDataTypeStr=int16  SampleTime=1e-08  SaturateOnIntegerOverflow=off  InputSameDT=off
  Resett_switch2 : Switch  Criteria=u2 ~= 0  Threshold=double(0)  OutDataTypeStr=int16  SampleTime=1e-08  SaturateOnIntegerOverflow=off  InputSameDT=off
  rd_{0..6} (7 alike) : Delay  DelayLength=double(1)  InitialCondition=0  SampleTime=1e-08
  reset_old_switch1 : Switch  Criteria=u2 ~= 0  Threshold=double(0)  OutDataTypeStr=int16  SampleTime=1e-08  SaturateOnIntegerOverflow=off  InputSameDT=off
  speed_old_switch1 : Switch  Criteria=u2 ~= 0  Threshold=double(0)  OutDataTypeStr=int16  SampleTime=1e-08  SaturateOnIntegerOverflow=off  InputSameDT=off
  count : Outport  SampleTime=1e-08  VectorParamsAs1DForOutWhenUnconnected=off
  wires:
  Edge/1 -> speed_old_switch1/2
  IncsPerTurn/1 -> rd_0/1
  Constant1/1 -> Resett_switch1/1, Resett_switch2/1
  Constant2/1 -> rd_3/1
  Constant3/1 -> speed_old_switch1/3
  Constant4/1 -> Reset_when_overflow/1
  Reset_when_overflow/1 -> rd_1/1
  reset_old_switch1/1 -> rd_6/1, count/1
  speed_old_switch1/1 -> Add1/1
  Resett_switch2/1 -> rd_4/1
  Add1/1 -> Resett_switch2/3
  Relational Operator/1 -> rd_5/1
  Resett_switch1/1 -> Add1/2, Relational Operator/1, reset_old_switch1/1
  rd_0/1 -> Reset_when_overflow/2
  rd_3/1 -> speed_old_switch1/1
  rd_6/1 -> reset_old_switch1/3
  rd_4/1 -> Resett_switch1/3
  rd_1/1 -> Relational Operator/2
  rd_5/1 -> Resett_switch1/2
  Reset/1 -> rd_2/1
  rd_2/1 -> reset_old_switch1/2, Resett_switch2/2

== system gm_inc_enc_v26/IncEnc_V26/digital_filter ==
  A : Inport  OutDataTypeStr=boolean  PortDimensions=1  SampleTime=1e-08
  AND : Logic  Inputs=3  AllPortsSameDT=off  OutDataTypeStr=boolean  SampleTime=1e-08
  AND1 : Logic  Inputs=3  AllPortsSameDT=off  OutDataTypeStr=boolean  SampleTime=1e-08
  NOT : Logic  Operator=NOT  Inputs=1  AllPortsSameDT=off  OutDataTypeStr=boolean  SampleTime=1e-08
  NOT1 : Logic  Operator=NOT  Inputs=1  AllPortsSameDT=off  OutDataTypeStr=boolean  SampleTime=1e-08
  NOT2 : Logic  Operator=NOT  Inputs=1  AllPortsSameDT=off  OutDataTypeStr=boolean  SampleTime=1e-08
  Subsystem1 : Subsystem
  rd_0 : Delay  DelayLength=double(2)  InitialCondition=0  SampleTime=1e-08
  rd_{1..4} (4 alike) : Delay  DelayLength=double(1)  InitialCondition=0  SampleTime=1e-08
  Q : Outport  SampleTime=1e-08
  wires:
  AND/1 -> rd_3/1
  AND1/1 -> Subsystem1/2(R)
  NOT/1 -> AND1/1
  NOT1/1 -> AND1/2
  NOT2/1 -> AND1/3
  Subsystem1/1(Q) -> Q/1
  rd_3/1 -> Subsystem1/1(S)
  A/1 -> rd_0/1
  rd_0/1 -> AND/1, rd_1/1
  rd_1/1 -> AND/2, NOT/1, rd_2/1
  rd_2/1 -> AND/3, NOT1/1, rd_4/1
  rd_4/1 -> NOT2/1
